simulink model "test_ads5296_fmca_r2_fmcb_r2_clk0"  (R2019a)
settings: Solver=FixedStepAuto  StartTime=0.0  StopTime=10.0  RelTol=1e-3
libraries: xbsIndex_r4 x3583, casper_library_misc x2, xps_library x1
(part 1 of 35)
settings Model: Creator=jackh  LastModifiedBy=jackh
settings DataIOCC: ReturnWorkspaceOutputs=off
settings DebuggingCC: PregeneratedLibrarySubsystemCodeDiagnostic=none  ArithmeticOperatorsInVariantConditions=warning
settings SFSimCC: SimUseLocalCustomCode=off
settings RTWCC: RTWUseLocalCustomCode=off

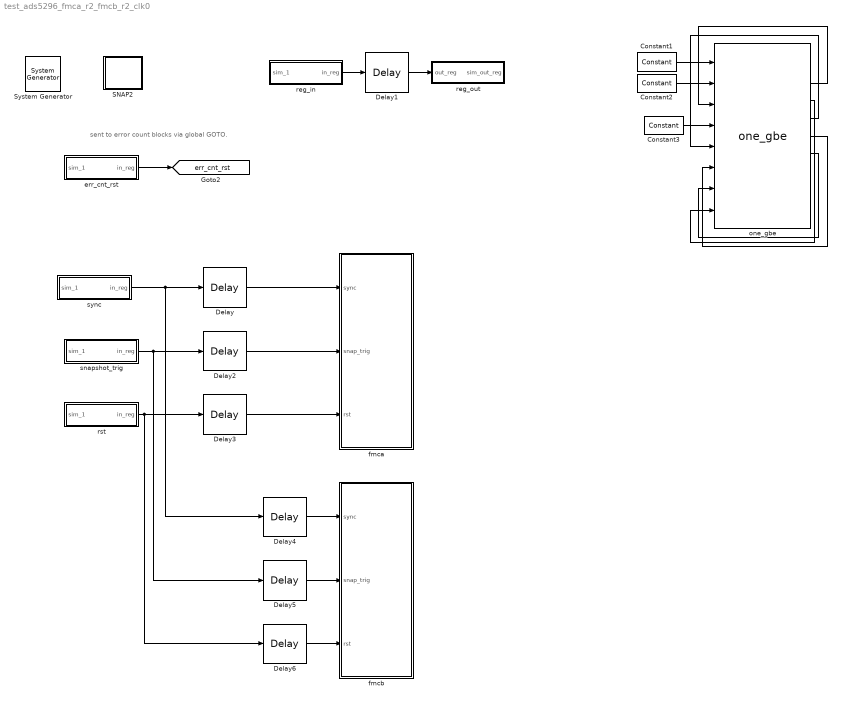
== system test_ads5296_fmca_r2_fmcb_r2_clk0 ==
  note: sent to error count blocks via global GOTO.
  " System Generator" : xbsIndex_r4/ System Generator  Tag=genX  xilinxfamily=kintexu  part=xcku115  speed=-2-e  package=flvf1924  synthesis_tool=XST  clock_wrapper=Clock Enables  directory=/home/jackh/src/caltech-lwa/test_models/ads5296_snap2_clkswitch_c/sysgen  proj_type=Vivado  Synth_file=Vivado Synthesis Defaults  Impl_file=Vivado Implementation Defaults  testbench=off  simulink_period=1  sysclk_period=5  dcm_input_clock_period=10  incr_netlist=off  trim_vbits=Everywhere in SubSystem  dbl_ovrd=According to Block Masks  core_generation=According to Block Masks  run_coregen=off  deprecated_control=off  eval_field=0  block_type=sysgen
  Constant1 : xbsIndex_r4/Constant  const=0  gui_display_data_type=Boolean  arith_type=Boolean  n_bits=16  bin_pt=14  preci_type=Single  exp_width=8  frac_width=24  explicit_period=on  period=1  equ=P=C  opselect=C  inp2=PCIN>>17  opr=+  inp1=P  carry=CIN  dbl_ovrd=off  block_type=constant
  Constant2 : xbsIndex_r4/Constant  const=0  gui_display_data_type=Boolean  arith_type=Boolean  n_bits=16  bin_pt=14  preci_type=Single  exp_width=8  frac_width=24  explicit_period=on  period=1  equ=P=C  opselect=C  inp2=PCIN>>17  opr=+  inp1=P  carry=CIN  dbl_ovrd=off  block_type=constant
  Constant3 : xbsIndex_r4/Constant  const=0  gui_display_data_type=Boolean  arith_type=Boolean  n_bits=16  bin_pt=14  preci_type=Single  exp_width=8  frac_width=24  explicit_period=on  period=1  equ=P=C  opselect=C  inp2=PCIN>>17  opr=+  inp1=P  carry=CIN  dbl_ovrd=off  block_type=constant
  Delay{,1..6} (7 alike) : xbsIndex_r4/Delay  rst=off  infoeditControl=Selection of Reset will increase slice count due to use of real FFs and instead of SRLs  en=off  latency=1  reg_retiming=off  dbl_ovrd=off  block_type=delay
  SNAP2 : Subsystem  Tag=xps:xsg  mask(xsg core config){hw_sys=SNAP2_v2:xcku115, clk_src=adc0_clk, clk_rate=200, use_microblaze=on, sample_period=1, synthesis_tool=XST}
      mask prompts: hw_sys "Hardware Platform"; clk_src "User IP Clock source"; clk_rate "User IP Clock Rate (MHz)"; use_microblaze "Use Microblaze controller?"; sample_period "Sample Period"; synthesis_tool "Synthesis Tool:"
      mask help:
      | The XSG Core Config block is used to configure the System Generator design
      | for the casper_xps toolflow. Settings here are used to configure the
      | Xilinx System Generator block parameters automatically, and control toolflow
      | script  execution. It needs to be at the top level of all designs being compiled
      | with the casper_xps toolflow.
      mask init:
      | xps_xsg_snap2_conf_mask;
      mask Help: eval('xlWeb([getenv(''MLIB_ROOT''), ''\doc\html\sys_xsg_core_config\sys_xsg_core_config.html''])')
      mask TypeOptions hw_sys: SNAP2_v1:xcku115 | SNAP2_v2:xcku115
      mask TypeOptions clk_src: sys_clk | clk_250MHz | adc0_clk | adc1_clk
      mask TypeOptions synthesis_tool: Leonardo Spectrum | Synplify | Synplify Pro | XST
      mask Display: fprintf(['SNAP2']);
  err_cnt_rst : Subsystem  Tag=xps:sw_reg  AncestorBlock=xps_library/Memory/software_register  mask(swreg){io_dir=From Processor, io_delay=0, init_val=0, sample_period=1, names=reg, bitwidths=1, bin_pts=0, arith_types=2, sim_port=on, show_format=on}
      mask prompts: io_dir "I/O direction"; io_delay "I/O delay"; init_val "Initial Value"; sample_period "Sample period"; names "Bitfield names [msb...lsb]"; bitwidths "Bitfield widths"; bin_pts "Bitfield binary pts"; arith_types "Bitfield types, ufix=0, fix=1, bool=2"; sim_port "Provide sim input/output?"; show_format "Print format string?"
      mask help: A 32-bit software-accessible register. Can be divided into bitfields of varying widths and types using the fields in the block mask.
      mask init:
      | swreg_init(gcb)
      settings: AttributesFormatString=1input:b = 1 bits
      mask TypeOptions io_dir: To Processor | From Processor
      mask Callback io_dir:
      | mask_enables = get_param(gcb, 'MaskEnables');
      | mask_names = get_param(gcb, 'MaskNames');
      | if strcmp(get_param(gcb, 'io_dir'), 'To Processor'),
      |     mask_enables{ismember(mask_names, 'sample_period')} = 'off';
      | else
      |     mask_enables{ismember(mask_names, 'sample_period')} = 'on';
      | end
      | set_param(gcb, 'MaskEnables', mask_enables);
      mask DialogControl ParameterTabVar0 Prompt: Setup
  fmca : Subsystem  mask{fmc_port=0, fmc_clock=0, board_version=2}
      mask prompts: fmc_port "FMC port"; fmc_clock "Use clock from which FMC"; board_version "Board version"
  fmcb : Subsystem  mask{fmc_port=1, fmc_clock=0, board_version=2}
      mask prompts: fmc_port "FMC port"; fmc_clock "Use clock from which FMC"; board_version "Board version"
  one_gbe : xps_library/IO/one_gbe  Tag=xps:onegbe  local_en=on  dis_cpu_rx=off  dis_cpu_tx=off  cpu_promiscuous=on  local_mac=hex2dec('123456789abc')  local_ip=hex2dec('c0a8290a')  local_port=4321  local_gateway=1
      settings: SourceProductName=CASPER XPS Blockset
  reg_in : Subsystem  Tag=xps:sw_reg  AncestorBlock=xps_library/Memory/software_register  mask(swreg){io_dir=From Processor, io_delay=0, init_val=0, sample_period=1, names=reg, bitwidths=10, bin_pts=9, arith_types=1, sim_port=on, show_format=on}
      mask prompts: io_dir "I/O direction"; io_delay "I/O delay"; init_val "Initial Value"; sample_period "Sample period"; names "Bitfield names [msb...lsb]"; bitwidths "Bitfield widths"; bin_pts "Bitfield binary pts"; arith_types "Bitfield types, ufix=0, fix=1, bool=2"; sim_port "Provide sim input/output?"; show_format "Print format string?"
      mask help: A 32-bit software-accessible register. Can be divided into bitfields of varying widths and types using the fields in the block mask.
      mask init:
      | swreg_init(gcb)
      settings: AttributesFormatString=1input:f10.9 = 10 bits
      mask TypeOptions io_dir: To Processor | From Processor
      mask Callback io_dir:
      | mask_enables = get_param(gcb, 'MaskEnables');
      | mask_names = get_param(gcb, 'MaskNames');
      | if strcmp(get_param(gcb, 'io_dir'), 'To Processor'),
      |     mask_enables{ismember(mask_names, 'sample_period')} = 'off';
      | else
      |     mask_enables{ismember(mask_names, 'sample_period')} = 'on';
      | end
      | set_param(gcb, 'MaskEnables', mask_enables);
      mask DialogControl ParameterTabVar0 Prompt: Setup
  reg_out : Subsystem  Tag=xps:sw_reg  AncestorBlock=xps_library/Memory/software_register  mask(swreg){io_dir=To Processor, io_delay=0, init_val=0, sample_period=1, names=reg, bitwidths=10, bin_pts=9, arith_types=1, sim_port=on, show_format=on}
      mask prompts: io_dir "I/O direction"; io_delay "I/O delay"; init_val "Initial Value"; sample_period "Sample period"; names "Bitfield names [msb...lsb]"; bitwidths "Bitfield widths"; bin_pts "Bitfield binary pts"; arith_types "Bitfield types, ufix=0, fix=1, bool=2"; sim_port "Provide sim input/output?"; show_format "Print format string?"
      mask help: A 32-bit software-accessible register. Can be divided into bitfields of varying widths and types using the fields in the block mask.
      mask init:
      | swreg_init(gcb)
      settings: AttributesFormatString=1output:f10.9 = 10 bits
      mask TypeOptions io_dir: To Processor | From Processor
      mask Callback io_dir:
      | mask_enables = get_param(gcb, 'MaskEnables');
      | mask_names = get_param(gcb, 'MaskNames');
      | if strcmp(get_param(gcb, 'io_dir'), 'To Processor'),
      |     mask_enables{ismember(mask_names, 'sample_period')} = 'off';
      | else
      |     mask_enables{ismember(mask_names, 'sample_period')} = 'on';
      | end
      | set_param(gcb, 'MaskEnables', mask_enables);
      mask DialogControl ParameterTabVar0 Prompt: Setup
  rst : Subsystem  Tag=xps:sw_reg  AncestorBlock=xps_library/Memory/software_register  mask(swreg){io_dir=From Processor, io_delay=0, init_val=0, sample_period=1, names=reg, bitwidths=1, bin_pts=0, arith_types=2, sim_port=on, show_format=on}
      mask prompts: io_dir "I/O direction"; io_delay "I/O delay"; init_val "Initial Value"; sample_period "Sample period"; names "Bitfield names [msb...lsb]"; bitwidths "Bitfield widths"; bin_pts "Bitfield binary pts"; arith_types "Bitfield types, ufix=0, fix=1, bool=2"; sim_port "Provide sim input/output?"; show_format "Print format string?"
      mask help: A 32-bit software-accessible register. Can be divided into bitfields of varying widths and types using the fields in the block mask.
      mask init:
      | swreg_init(gcb)
      settings: AttributesFormatString=1input:b = 1 bits
      mask TypeOptions io_dir: To Processor | From Processor
      mask Callback io_dir:
      | mask_enables = get_param(gcb, 'MaskEnables');
      | mask_names = get_param(gcb, 'MaskNames');
      | if strcmp(get_param(gcb, 'io_dir'), 'To Processor'),
      |     mask_enables{ismember(mask_names, 'sample_period')} = 'off';
      | else
      |     mask_enables{ismember(mask_names, 'sample_period')} = 'on';
      | end
      | set_param(gcb, 'MaskEnables', mask_enables);
      mask DialogControl ParameterTabVar0 Prompt: Setup
  snapshot_trig : Subsystem  Tag=xps:sw_reg  AncestorBlock=xps_library/Memory/software_register  mask(swreg){io_dir=From Processor, io_delay=0, init_val=0, sample_period=1, names=reg, bitwidths=1, bin_pts=0, arith_types=2, sim_port=on, show_format=on}
      mask prompts: io_dir "I/O direction"; io_delay "I/O delay"; init_val "Initial Value"; sample_period "Sample period"; names "Bitfield names [msb...lsb]"; bitwidths "Bitfield widths"; bin_pts "Bitfield binary pts"; arith_types "Bitfield types, ufix=0, fix=1, bool=2"; sim_port "Provide sim input/output?"; show_format "Print format string?"
      mask help: A 32-bit software-accessible register. Can be divided into bitfields of varying widths and types using the fields in the block mask.
      mask init:
      | swreg_init(gcb)
      settings: AttributesFormatString=1input:b = 1 bits
      mask TypeOptions io_dir: To Processor | From Processor
      mask Callback io_dir:
      | mask_enables = get_param(gcb, 'MaskEnables');
      | mask_names = get_param(gcb, 'MaskNames');
      | if strcmp(get_param(gcb, 'io_dir'), 'To Processor'),
      |     mask_enables{ismember(mask_names, 'sample_period')} = 'off';
      | else
      |     mask_enables{ismember(mask_names, 'sample_period')} = 'on';
      | end
      | set_param(gcb, 'MaskEnables', mask_enables);
      mask DialogControl ParameterTabVar0 Prompt: Setup
  sync : Subsystem  Tag=xps:sw_reg  AncestorBlock=xps_library/Memory/software_register  mask(swreg){io_dir=From Processor, io_delay=0, init_val=0, sample_period=1, names=reg, bitwidths=1, bin_pts=0, arith_types=2, sim_port=on, show_format=on}
      mask prompts: io_dir "I/O direction"; io_delay "I/O delay"; init_val "Initial Value"; sample_period "Sample period"; names "Bitfield names [msb...lsb]"; bitwidths "Bitfield widths"; bin_pts "Bitfield binary pts"; arith_types "Bitfield types, ufix=0, fix=1, bool=2"; sim_port "Provide sim input/output?"; show_format "Print format string?"
      mask help: A 32-bit software-accessible register. Can be divided into bitfields of varying widths and types using the fields in the block mask.
      mask init:
      | swreg_init(gcb)
      settings: AttributesFormatString=1input:b = 1 bits
      mask TypeOptions io_dir: To Processor | From Processor
      mask Callback io_dir:
      | mask_enables = get_param(gcb, 'MaskEnables');
      | mask_names = get_param(gcb, 'MaskNames');
      | if strcmp(get_param(gcb, 'io_dir'), 'To Processor'),
      |     mask_enables{ismember(mask_names, 'sample_period')} = 'off';
      | else
      |     mask_enables{ismember(mask_names, 'sample_period')} = 'on';
      | end
      | set_param(gcb, 'MaskEnables', mask_enables);
      mask DialogControl ParameterTabVar0 Prompt: Setup
  tag scope: err_cnt_rst=global
  wires:
  reg_in/1(in_reg) -> Delay1/1
  Delay1/1 -> reg_out/1(out_reg)
  Constant1/1 -> one_gbe/1
  Constant2/1 -> one_gbe/2
  one_gbe/3 -> one_gbe/3
  Constant3/1 -> one_gbe/4
  one_gbe/5 -> one_gbe/5
  one_gbe/6 -> one_gbe/6
  one_gbe/7 -> one_gbe/7
  one_gbe/4 -> one_gbe/8
  err_cnt_rst/1(in_reg) -> [err_cnt_rst]
  sync/1(in_reg) -> Delay4/1, Delay/1
  snapshot_trig/1(in_reg) -> Delay5/1, Delay2/1
  rst/1(in_reg) -> Delay6/1, Delay3/1
  Delay/1 -> fmca/1(sync)
  Delay2/1 -> fmca/2(snap_trig)
  Delay3/1 -> fmca/3(rst)
  Delay4/1 -> fmcb/1(sync)
  Delay5/1 -> fmcb/2(snap_trig)
  Delay6/1 -> fmcb/3(rst)

== system test_ads5296_fmca_r2_fmcb_r2_clk0/SNAP2 ==

== system test_ads5296_fmca_r2_fmcb_r2_clk0/err_cnt_rst ==
  sim_1 : Inport
  convert1_1 : DataTypeConversion  OutDataTypeStr=fixdt('ufix1_En0')  LockScale=on
  convert2_1 : DataTypeConversion  OutDataTypeStr=fixdt('ufix1_En0')  ConvertRealWorld=Stored Integer (SI)  LockScale=on
  gain_1 : Gain
  io_delay : xbsIndex_r4/Delay  rst=off  infoeditControl=Selection of Reset will increase slice count due to use of real FFs and instead of SRLs  en=off  latency=0  reg_retiming=on  dbl_ovrd=off  block_type=delay
  slice_reg : xbsIndex_r4/Slice  nbits=1  boolean_output=on  mode=Lower Bit Location + Width  bit1=0  base1=MSB of Input  bit0=0  base0=LSB of Input  dbl_ovrd=off  block_type=slice
  test_ads5296_fmca_r2_fmcb_r2_clk0_err_cnt_rst_user_data_out : xbsIndex_r4/Gateway In  gui_display_data_type=Fixed-point  arith_type=Unsigned  n_bits=32  bin_pt=0  preci_type=Single  exp_width=8  frac_width=24  rows=1  columns=1  quantization="Round  (unbiased: +/- Inf)"  overflow=Saturate  period=1  UseAsADC=off  ADCChannel='1'  interface=None  automatic_assignment=on  address_offset=hex2dec('00')  intf_name=''  intf_description=''  default_value=0  timing_constraint=None  locs_specified=off  LOCs={}  io_standard={}  inherit_from_input=off  hdl_port=on  dbl_ovrd=off  block_type=gatewayin
  in_reg : Outport
  wires:
  test_ads5296_fmca_r2_fmcb_r2_clk0_err_cnt_rst_user_data_out/1 -> io_delay/1
  sim_1/1 -> convert1_1/1
  convert1_1/1 -> convert2_1/1
  convert2_1/1 -> gain_1/1
  gain_1/1 -> test_ads5296_fmca_r2_fmcb_r2_clk0_err_cnt_rst_user_data_out/1
  io_delay/1 -> slice_reg/1
  slice_reg/1 -> in_reg/1

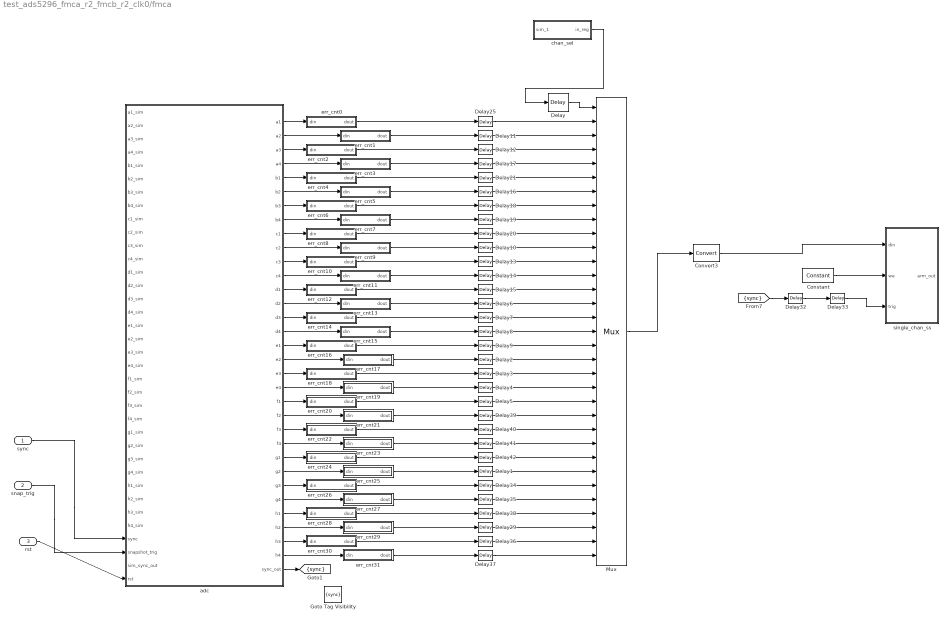
== system test_ads5296_fmca_r2_fmcb_r2_clk0/fmca ==
  sync : Inport
  snap_trig : Inport  Port=2
  rst : Inport  Port=3
  Constant : xbsIndex_r4/Constant  const=1  gui_display_data_type=Boolean  arith_type=Boolean  n_bits=16  bin_pt=14  preci_type=Single  exp_width=8  frac_width=24  explicit_period=on  period=1  equ=P=C  opselect=C  inp2=PCIN>>17  opr=+  inp1=P  carry=CIN  dbl_ovrd=off  block_type=constant
  Convert3 : xbsIndex_r4/Convert  gui_display_data_type=Fixed-point  arith_type="Signed  (2's comp)"  n_bits=16  bin_pt=15  float_type=Single  exp_bits=8  fraction_bits=24  quantization=Truncate  overflow=Wrap  en=off  latency=0  pipeline=off  dbl_ovrd=off  block_type=convert
  Delay : xbsIndex_r4/Delay  rst=off  infoeditControl=Selection of Reset will increase slice count due to use of real FFs and instead of SRLs  en=off  latency=6  reg_retiming=on  dbl_ovrd=off  block_type=delay
  Delay{1..21,25,29,32,34..42} (33 alike) : xbsIndex_r4/Delay  rst=off  infoeditControl=Selection of Reset will increase slice count due to use of real FFs and instead of SRLs  en=off  latency=2  reg_retiming=on  dbl_ovrd=off  block_type=delay
  Delay33 : xbsIndex_r4/Delay  rst=off  infoeditControl=Selection of Reset will increase slice count due to use of real FFs and instead of SRLs  en=off  latency=4  reg_retiming=on  dbl_ovrd=off  block_type=delay
  Goto Tag Visibility : GotoTagVisibility  GotoTag=sync
  Mux : xbsIndex_r4/Mux  inputs=32  en=off  latency=4  precision=Full  arith_type=Unsigned  n_bits=16  bin_pt=14  quantization=Truncate  overflow=Wrap  dbl_ovrd=off  block_type=mux
  adc : Subsystem  Tag=xps:ads5296x4  mask(ADS5296x4){board_count=2, sample_rate=200, port=fmc_port, clockport=fmc_clock, version=board_version}
      mask prompts: board_count "Number of quad-chip ADC Boards"; sample_rate "Sample Rate"; port "Which FMC port?"; clockport "Use clock from which FMC board?"; version "Which ADC board version?"
      mask help: 16-input ADC based on the TI ADS5296 chip.
      mask init:
      | % Only board_count is needed by init function
      | ads5296x4_init(gcb, ...
      |     'board_count', board_count);
      mask TypeOptions board_count: 1 | 2 | 3 | 4
  chan_sel : Subsystem  Tag=xps:sw_reg  AncestorBlock=xps_library/Memory/software_register  mask(swreg){io_dir=From Processor, io_delay=0, init_val=0, sample_period=1, names=reg, bitwidths=5, bin_pts=0, arith_types=0, sim_port=on, show_format=on}
      mask prompts: io_dir "I/O direction"; io_delay "I/O delay"; init_val "Initial Value"; sample_period "Sample period"; names "Bitfield names [msb...lsb]"; bitwidths "Bitfield widths"; bin_pts "Bitfield binary pts"; arith_types "Bitfield types, ufix=0, fix=1, bool=2"; sim_port "Provide sim input/output?"; show_format "Print format string?"
      mask help: A 32-bit software-accessible register. Can be divided into bitfields of varying widths and types using the fields in the block mask.
      mask init:
      | swreg_init(gcb)
      settings: AttributesFormatString=1input:uf5.0 = 5 bits
      mask TypeOptions io_dir: To Processor | From Processor
      mask Callback io_dir:
      | mask_enables = get_param(gcb, 'MaskEnables');
      | mask_names = get_param(gcb, 'MaskNames');
      | if strcmp(get_param(gcb, 'io_dir'), 'To Processor'),
      |     mask_enables{ismember(mask_names, 'sample_period')} = 'off';
      | else
      |     mask_enables{ismember(mask_names, 'sample_period')} = 'on';
      | end
      | set_param(gcb, 'MaskEnables', mask_enables);
      mask DialogControl ParameterTabVar0 Prompt: Setup
  err_cnt0 : Subsystem  VariantControl=Variant1
  err_cnt1 : Subsystem  VariantControl=Variant1
  err_cnt10 : Subsystem  VariantControl=Variant1
  err_cnt11 : Subsystem  VariantControl=Variant1
  err_cnt12 : Subsystem  VariantControl=Variant1
  err_cnt13 : Subsystem  VariantControl=Variant1
  err_cnt14 : Subsystem  VariantControl=Variant1
  err_cnt15 : Subsystem  VariantControl=Variant1
  err_cnt16 : Subsystem  VariantControl=Variant1
  err_cnt17 : Subsystem  VariantControl=Variant1
  err_cnt18 : Subsystem  VariantControl=Variant1
  err_cnt19 : Subsystem  VariantControl=Variant1
  err_cnt2 : Subsystem  VariantControl=Variant1
  err_cnt20 : Subsystem  VariantControl=Variant1
  err_cnt21 : Subsystem  VariantControl=Variant1
  err_cnt22 : Subsystem  VariantControl=Variant1
  err_cnt23 : Subsystem  VariantControl=Variant1
  err_cnt24 : Subsystem  VariantControl=Variant1
  err_cnt25 : Subsystem  VariantControl=Variant1
  err_cnt26 : Subsystem  VariantControl=Variant1
  err_cnt27 : Subsystem  VariantControl=Variant1
  err_cnt28 : Subsystem  VariantControl=Variant1
  err_cnt29 : Subsystem  VariantControl=Variant1
  err_cnt3 : Subsystem  VariantControl=Variant1
  err_cnt30 : Subsystem  VariantControl=Variant1
  err_cnt31 : Subsystem  VariantControl=Variant1
  err_cnt4 : Subsystem  VariantControl=Variant1
  err_cnt5 : Subsystem  VariantControl=Variant1
  err_cnt6 : Subsystem  VariantControl=Variant1
  err_cnt7 : Subsystem  VariantControl=Variant1
  err_cnt8 : Subsystem  VariantControl=Variant1
  err_cnt9 : Subsystem  VariantControl=Variant1
  single_chan_ss : Subsystem  Tag=casper:snapshot  AncestorBlock=casper_library_scopes/snapshot  mask(snapshot){storage=bram, dram_dimm=2, dram_clock=250, nsamples=16, data_width=16, offset=off, circap=off, value=off, ext_arm=off, ext_circ=off, provide_outputs=on, use_dsp48=off}
      mask prompts: storage "Storage medium"; dram_dimm "DRAM dimm"; dram_clock "DRAM clock rate"; nsamples "Number of Samples (2^?)"; data_width "Data width"; offset "Start delay support"; circap "Circular capture support"; value "Extra value capture support"; ext_arm "External arm support"; ext_circ "External circular capture support"; provide_outputs "Provide outputs"; use_dsp48 "Use DSP48s to implement counters"
      mask help:
      | Standard snap block, but with the following optional extras;
      |  1) Optionally delay the fabric trigger by a user-specified number of valids.
      |  2) Capture continuously after a trigger until a stop pulse is received. Data is captured into BRAM continuously, with old data being overwritten until a stop command is received. Then stop capturing when memory is filled. This enables you to get some data before and some data after the stop pulse. Use the 'tr_en_cnt' register to determine where you are in your vector. 'Addr' register's MSb now indicates 'busy capturing'.
      |  3) Optionally capture a value on an input port to a register at the same time as the first data sample.
      |  4) Implement counters using DSP48Es to save resources.
      mask init:
      | snapshot_init(gcb, ...
      |     'storage', storage, ...
      |     'dram_dimm', dram_dimm, ...
      |     'dram_clock', dram_clock, ...
      |     'nsamples', nsamples, ...
      |     'data_width', data_width, ...
      |     'offset', offset, ...
      |     'circap', circap, ...
      |     'value', value, ...
      |     'ext_arm', ext_arm, ...
      |     'ext_circ', ext_circ, ...
      |     'provide_outputs', 'off', ...
      |     'use_dsp48', use_dsp48);
      settings: AttributesFormatString=|
      | 16 wide, 65536 deep
      | debugID: 35264124
      mask TypeOptions storage: bram | dram
      mask Callback storage: snapshot_callback();
      mask TypeOptions dram_dimm: 1 | 2 | 3 | 4
      mask TypeOptions dram_clock: 200 | 250 | 266 | 300 | 333
      mask TypeOptions data_width: 8 | 16 | 32 | 64 | 128
  tag scope: sync=scoped
  wires:
  adc/16(d4) -> err_cnt15/1(din)
  adc/13(d1) -> err_cnt12/1(din)
  snap_trig/1 -> adc/34(snapshot_trig)
  adc/24(f4) -> err_cnt23/1(din)
  adc/2(a2) -> err_cnt1/1(din)
  adc/1(a1) -> err_cnt0/1(din)
  adc/23(f3) -> err_cnt22/1(din)
  Delay32/1 -> Delay33/1
  adc/4(a4) -> err_cnt3/1(din)
  adc/31(h3) -> err_cnt30/1(din)
  adc/27(g3) -> err_cnt26/1(din)
  adc/6(b2) -> err_cnt5/1(din)
  Mux/1 -> Convert3/1
  ? -> adc/35(sim_sync_out)
  adc/3(a3) -> err_cnt2/1(din)
  Delay36/1 -> Mux/32
  adc/32(h4) -> err_cnt31/1(din)
  Convert3/1 -> single_chan_ss/1(din)
  adc/33(sync_out) -> [sync]
  adc/5(b1) -> err_cnt4/1(din)
  adc/25(g1) -> err_cnt24/1(din)
  adc/18(e2) -> err_cnt17/1(din)
  adc/8(b4) -> err_cnt7/1(din)
  adc/10(c2) -> err_cnt9/1(din)
  Constant/1 -> single_chan_ss/2(we)
  Delay29/1 -> Mux/31
  adc/20(e4) -> err_cnt19/1(din)
  Delay37/1 -> Mux/33
  chan_sel/1(in_reg) -> Delay/1
  adc/12(c4) -> err_cnt11/1(din)
  rst/1 -> adc/36(rst)
  adc/26(g2) -> err_cnt25/1(din)
  sync/1 -> adc/33(sync)
  adc/14(d2) -> err_cnt13/1(din)
  adc/11(c3) -> err_cnt10/1(din)
  [sync] -> Delay32/1
  adc/22(f2) -> err_cnt21/1(din)
  adc/7(b3) -> err_cnt6/1(din)
  adc/29(h1) -> err_cnt28/1(din)
  adc/19(e3) -> err_cnt18/1(din)
  adc/15(d3) -> err_cnt14/1(din)
  adc/9(c1) -> err_cnt8/1(din)
  Delay/1 -> Mux/1
  adc/21(f1) -> err_cnt20/1(din)
  adc/30(h2) -> err_cnt29/1(din)
  adc/28(g4) -> err_cnt27/1(din)
  Delay33/1 -> single_chan_ss/3(trig)
  err_cnt31/1(dout) -> Delay37/1
  adc/17(e1) -> err_cnt16/1(din)
  err_cnt29/1(dout) -> Delay29/1
  err_cnt30/1(dout) -> Delay36/1
  err_cnt26/1(dout) -> Delay34/1
  err_cnt25/1(dout) -> Delay1/1
  err_cnt27/1(dout) -> Delay35/1
  err_cnt28/1(dout) -> Delay38/1
  err_cnt24/1(dout) -> Delay42/1
  err_cnt23/1(dout) -> Delay41/1
  err_cnt21/1(dout) -> Delay39/1
  err_cnt22/1(dout) -> Delay40/1
  err_cnt14/1(dout) -> Delay7/1
  err_cnt13/1(dout) -> Delay6/1
  err_cnt15/1(dout) -> Delay8/1
  err_cnt16/1(dout) -> Delay9/1
  err_cnt20/1(dout) -> Delay5/1
  err_cnt19/1(dout) -> Delay4/1
  err_cnt17/1(dout) -> Delay2/1
  err_cnt18/1(dout) -> Delay3/1
  err_cnt2/1(dout) -> Delay12/1
  err_cnt1/1(dout) -> Delay11/1
  err_cnt3/1(dout) -> Delay17/1
  err_cnt4/1(dout) -> Delay21/1
  err_cnt0/1(dout) -> Delay25/1
  err_cnt6/1(dout) -> Delay18/1
  err_cnt5/1(dout) -> Delay16/1
  err_cnt7/1(dout) -> Delay19/1
  err_cnt8/1(dout) -> Delay20/1
  err_cnt12/1(dout) -> Delay15/1
  err_cnt11/1(dout) -> Delay14/1
  err_cnt9/1(dout) -> Delay10/1
  err_cnt10/1(dout) -> Delay13/1
  Delay25/1 -> Mux/2
  Delay11/1 -> Mux/3
  Delay12/1 -> Mux/4
  Delay17/1 -> Mux/5
  Delay21/1 -> Mux/6
  Delay16/1 -> Mux/7
  Delay18/1 -> Mux/8
  Delay19/1 -> Mux/9
  Delay20/1 -> Mux/10
  Delay10/1 -> Mux/11
  Delay13/1 -> Mux/12
  Delay14/1 -> Mux/13
  Delay15/1 -> Mux/14
  Delay6/1 -> Mux/15
  Delay7/1 -> Mux/16
  Delay8/1 -> Mux/17
  Delay9/1 -> Mux/18
  Delay2/1 -> Mux/19
  Delay3/1 -> Mux/20
  Delay4/1 -> Mux/21
  Delay5/1 -> Mux/22
  Delay39/1 -> Mux/23
  Delay40/1 -> Mux/24
  Delay41/1 -> Mux/25
  Delay42/1 -> Mux/26
  Delay1/1 -> Mux/27
  Delay34/1 -> Mux/28
  Delay35/1 -> Mux/29
  Delay38/1 -> Mux/30

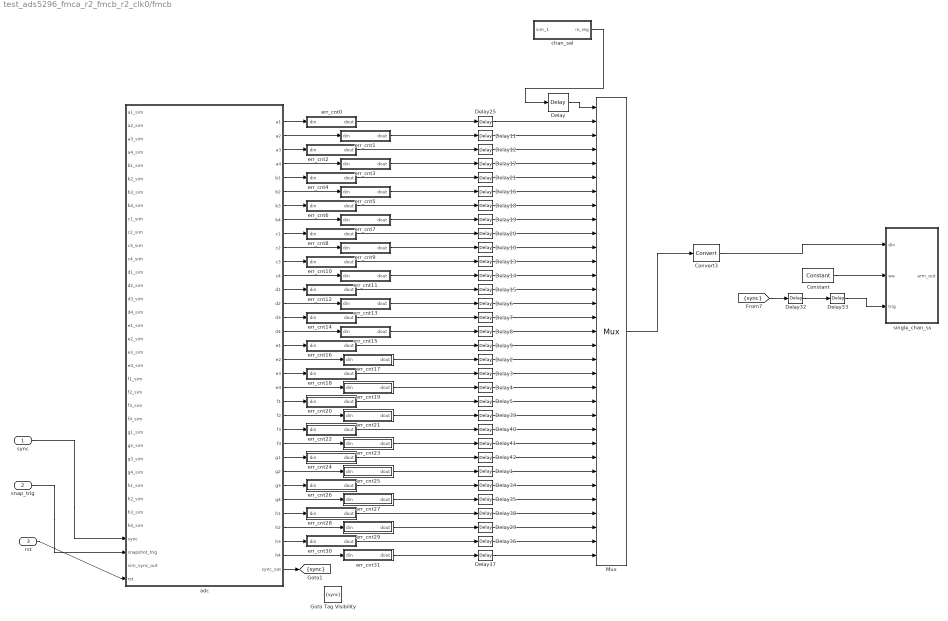
== system test_ads5296_fmca_r2_fmcb_r2_clk0/fmcb ==
  sync : Inport
  snap_trig : Inport  Port=2
  rst : Inport  Port=3
  Constant : xbsIndex_r4/Constant  const=1  gui_display_data_type=Boolean  arith_type=Boolean  n_bits=16  bin_pt=14  preci_type=Single  exp_width=8  frac_width=24  explicit_period=on  period=1  equ=P=C  opselect=C  inp2=PCIN>>17  opr=+  inp1=P  carry=CIN  dbl_ovrd=off  block_type=constant
  Convert3 : xbsIndex_r4/Convert  gui_display_data_type=Fixed-point  arith_type="Signed  (2's comp)"  n_bits=16  bin_pt=15  float_type=Single  exp_bits=8  fraction_bits=24  quantization=Truncate  overflow=Wrap  en=off  latency=0  pipeline=off  dbl_ovrd=off  block_type=convert
  Delay : xbsIndex_r4/Delay  rst=off  infoeditControl=Selection of Reset will increase slice count due to use of real FFs and instead of SRLs  en=off  latency=6  reg_retiming=on  dbl_ovrd=off  block_type=delay
  Delay{1..21,25,29,32,34..42} (33 alike) : xbsIndex_r4/Delay  rst=off  infoeditControl=Selection of Reset will increase slice count due to use of real FFs and instead of SRLs  en=off  latency=2  reg_retiming=on  dbl_ovrd=off  block_type=delay
  Delay33 : xbsIndex_r4/Delay  rst=off  infoeditControl=Selection of Reset will increase slice count due to use of real FFs and instead of SRLs  en=off  latency=4  reg_retiming=on  dbl_ovrd=off  block_type=delay
  Goto Tag Visibility : GotoTagVisibility  GotoTag=sync
  Mux : xbsIndex_r4/Mux  inputs=32  en=off  latency=4  precision=Full  arith_type=Unsigned  n_bits=16  bin_pt=14  quantization=Truncate  overflow=Wrap  dbl_ovrd=off  block_type=mux
  adc : Subsystem  Tag=xps:ads5296x4  mask(ADS5296x4){board_count=2, sample_rate=200, port=fmc_port, clockport=fmc_clock, version=board_version}
      mask prompts: board_count "Number of quad-chip ADC Boards"; sample_rate "Sample Rate"; port "Which FMC port?"; clockport "Use clock from which FMC board?"; version "Which ADC board version?"
      mask help: 16-input ADC based on the TI ADS5296 chip.
      mask init:
      | % Only board_count is needed by init function
      | ads5296x4_init(gcb, ...
      |     'board_count', board_count);
      mask TypeOptions board_count: 1 | 2 | 3 | 4
  chan_sel : Subsystem  Tag=xps:sw_reg  AncestorBlock=xps_library/Memory/software_register  mask(swreg){io_dir=From Processor, io_delay=0, init_val=0, sample_period=1, names=reg, bitwidths=5, bin_pts=0, arith_types=0, sim_port=on, show_format=on}
      mask prompts: io_dir "I/O direction"; io_delay "I/O delay"; init_val "Initial Value"; sample_period "Sample period"; names "Bitfield names [msb...lsb]"; bitwidths "Bitfield widths"; bin_pts "Bitfield binary pts"; arith_types "Bitfield types, ufix=0, fix=1, bool=2"; sim_port "Provide sim input/output?"; show_format "Print format string?"
      mask help: A 32-bit software-accessible register. Can be divided into bitfields of varying widths and types using the fields in the block mask.
      mask init:
      | swreg_init(gcb)
      settings: AttributesFormatString=1input:uf5.0 = 5 bits
      mask TypeOptions io_dir: To Processor | From Processor
      mask Callback io_dir:
      | mask_enables = get_param(gcb, 'MaskEnables');
      | mask_names = get_param(gcb, 'MaskNames');
      | if strcmp(get_param(gcb, 'io_dir'), 'To Processor'),
      |     mask_enables{ismember(mask_names, 'sample_period')} = 'off';
      | else
      |     mask_enables{ismember(mask_names, 'sample_period')} = 'on';
      | end
      | set_param(gcb, 'MaskEnables', mask_enables);
      mask DialogControl ParameterTabVar0 Prompt: Setup
  err_cnt0 : Subsystem  VariantControl=Variant1
  err_cnt1 : Subsystem  VariantControl=Variant1
  err_cnt10 : Subsystem  VariantControl=Variant1
  err_cnt11 : Subsystem  VariantControl=Variant1
  err_cnt12 : Subsystem  VariantControl=Variant1
  err_cnt13 : Subsystem  VariantControl=Variant1
  err_cnt14 : Subsystem  VariantControl=Variant1
  err_cnt15 : Subsystem  VariantControl=Variant1
  err_cnt16 : Subsystem  VariantControl=Variant1
  err_cnt17 : Subsystem  VariantControl=Variant1
  err_cnt18 : Subsystem  VariantControl=Variant1
  err_cnt19 : Subsystem  VariantControl=Variant1
  err_cnt2 : Subsystem  VariantControl=Variant1
  err_cnt20 : Subsystem  VariantControl=Variant1
  err_cnt21 : Subsystem  VariantControl=Variant1
  err_cnt22 : Subsystem  VariantControl=Variant1
  err_cnt23 : Subsystem  VariantControl=Variant1
  err_cnt24 : Subsystem  VariantControl=Variant1
  err_cnt25 : Subsystem  VariantControl=Variant1
  err_cnt26 : Subsystem  VariantControl=Variant1
  err_cnt27 : Subsystem  VariantControl=Variant1
  err_cnt28 : Subsystem  VariantControl=Variant1
  err_cnt29 : Subsystem  VariantControl=Variant1
  err_cnt3 : Subsystem  VariantControl=Variant1
  err_cnt30 : Subsystem  VariantControl=Variant1
  err_cnt31 : Subsystem  VariantControl=Variant1
  err_cnt4 : Subsystem  VariantControl=Variant1
  err_cnt5 : Subsystem  VariantControl=Variant1
  err_cnt6 : Subsystem  VariantControl=Variant1
  err_cnt7 : Subsystem  VariantControl=Variant1
  err_cnt8 : Subsystem  VariantControl=Variant1
  err_cnt9 : Subsystem  VariantControl=Variant1
  single_chan_ss : Subsystem  Tag=casper:snapshot  AncestorBlock=casper_library_scopes/snapshot  mask(snapshot){storage=bram, dram_dimm=2, dram_clock=250, nsamples=16, data_width=16, offset=off, circap=off, value=off, ext_arm=off, ext_circ=off, provide_outputs=on, use_dsp48=off}
      mask prompts: storage "Storage medium"; dram_dimm "DRAM dimm"; dram_clock "DRAM clock rate"; nsamples "Number of Samples (2^?)"; data_width "Data width"; offset "Start delay support"; circap "Circular capture support"; value "Extra value capture support"; ext_arm "External arm support"; ext_circ "External circular capture support"; provide_outputs "Provide outputs"; use_dsp48 "Use DSP48s to implement counters"
      mask help:
      | Standard snap block, but with the following optional extras;
      |  1) Optionally delay the fabric trigger by a user-specified number of valids.
      |  2) Capture continuously after a trigger until a stop pulse is received. Data is captured into BRAM continuously, with old data being overwritten until a stop command is received. Then stop capturing when memory is filled. This enables you to get some data before and some data after the stop pulse. Use the 'tr_en_cnt' register to determine where you are in your vector. 'Addr' register's MSb now indicates 'busy capturing'.
      |  3) Optionally capture a value on an input port to a register at the same time as the first data sample.
      |  4) Implement counters using DSP48Es to save resources.
      mask init: same as test_ads5296_fmca_r2_fmcb_r2_clk0/fmca/single_chan_ss
      settings: AttributesFormatString=|
      | 16 wide, 65536 deep
      | debugID: 35264124
      mask TypeOptions storage: bram | dram
      mask Callback storage: snapshot_callback();
      mask TypeOptions dram_dimm: 1 | 2 | 3 | 4
      mask TypeOptions dram_clock: 200 | 250 | 266 | 300 | 333
      mask TypeOptions data_width: 8 | 16 | 32 | 64 | 128
  tag scope: sync=scoped
  wires:
  Delay38/1 -> Mux/30
  Delay35/1 -> Mux/29
  Delay34/1 -> Mux/28
  Delay1/1 -> Mux/27
  Delay42/1 -> Mux/26
  Delay41/1 -> Mux/25
  Delay40/1 -> Mux/24
  Delay39/1 -> Mux/23
  Delay5/1 -> Mux/22
  Delay4/1 -> Mux/21
  Delay3/1 -> Mux/20
  Delay2/1 -> Mux/19
  Delay9/1 -> Mux/18
  Delay8/1 -> Mux/17
  Delay7/1 -> Mux/16
  Delay6/1 -> Mux/15
  Delay15/1 -> Mux/14
  Delay14/1 -> Mux/13
  Delay13/1 -> Mux/12
  Delay10/1 -> Mux/11
  Delay20/1 -> Mux/10
  Delay19/1 -> Mux/9
  Delay18/1 -> Mux/8
  Delay16/1 -> Mux/7
  Delay21/1 -> Mux/6
  Delay17/1 -> Mux/5
  Delay12/1 -> Mux/4
  Delay11/1 -> Mux/3
  Delay25/1 -> Mux/2
  err_cnt10/1(dout) -> Delay13/1
  err_cnt9/1(dout) -> Delay10/1
  err_cnt11/1(dout) -> Delay14/1
  err_cnt12/1(dout) -> Delay15/1
  err_cnt8/1(dout) -> Delay20/1
  err_cnt7/1(dout) -> Delay19/1
  err_cnt5/1(dout) -> Delay16/1
  err_cnt6/1(dout) -> Delay18/1
  err_cnt0/1(dout) -> Delay25/1
  err_cnt4/1(dout) -> Delay21/1
  err_cnt3/1(dout) -> Delay17/1
  err_cnt1/1(dout) -> Delay11/1
  err_cnt2/1(dout) -> Delay12/1
  err_cnt18/1(dout) -> Delay3/1
  err_cnt17/1(dout) -> Delay2/1
  err_cnt19/1(dout) -> Delay4/1
  err_cnt20/1(dout) -> Delay5/1
  err_cnt16/1(dout) -> Delay9/1
  err_cnt15/1(dout) -> Delay8/1
  err_cnt13/1(dout) -> Delay6/1
  err_cnt14/1(dout) -> Delay7/1
  err_cnt22/1(dout) -> Delay40/1
  err_cnt21/1(dout) -> Delay39/1
  err_cnt23/1(dout) -> Delay41/1
  err_cnt24/1(dout) -> Delay42/1
  err_cnt28/1(dout) -> Delay38/1
  err_cnt27/1(dout) -> Delay35/1
  err_cnt25/1(dout) -> Delay1/1
  err_cnt26/1(dout) -> Delay34/1
  err_cnt30/1(dout) -> Delay36/1
  err_cnt29/1(dout) -> Delay29/1
  adc/17(e1) -> err_cnt16/1(din)
  err_cnt31/1(dout) -> Delay37/1
  Delay33/1 -> single_chan_ss/3(trig)
  adc/28(g4) -> err_cnt27/1(din)
  adc/30(h2) -> err_cnt29/1(din)
  adc/21(f1) -> err_cnt20/1(din)
  Delay/1 -> Mux/1
  adc/9(c1) -> err_cnt8/1(din)
  adc/15(d3) -> err_cnt14/1(din)
  adc/19(e3) -> err_cnt18/1(din)
  adc/29(h1) -> err_cnt28/1(din)
  adc/7(b3) -> err_cnt6/1(din)
  adc/22(f2) -> err_cnt21/1(din)
  [sync] -> Delay32/1
  adc/11(c3) -> err_cnt10/1(din)
  adc/14(d2) -> err_cnt13/1(din)
  sync/1 -> adc/33(sync)
  adc/26(g2) -> err_cnt25/1(din)
  rst/1 -> adc/36(rst)
  adc/12(c4) -> err_cnt11/1(din)
  chan_sel/1(in_reg) -> Delay/1
  Delay37/1 -> Mux/33
  adc/20(e4) -> err_cnt19/1(din)
  Delay29/1 -> Mux/31
  Constant/1 -> single_chan_ss/2(we)
  adc/10(c2) -> err_cnt9/1(din)
  adc/8(b4) -> err_cnt7/1(din)
  adc/18(e2) -> err_cnt17/1(din)
  adc/25(g1) -> err_cnt24/1(din)
  adc/5(b1) -> err_cnt4/1(din)
  adc/33(sync_out) -> [sync]
  Convert3/1 -> single_chan_ss/1(din)
  adc/32(h4) -> err_cnt31/1(din)
  Delay36/1 -> Mux/32
  adc/3(a3) -> err_cnt2/1(din)
  ? -> adc/35(sim_sync_out)
  Mux/1 -> Convert3/1
  adc/6(b2) -> err_cnt5/1(din)
  adc/27(g3) -> err_cnt26/1(din)
  adc/31(h3) -> err_cnt30/1(din)
  adc/4(a4) -> err_cnt3/1(din)
  Delay32/1 -> Delay33/1
  adc/23(f3) -> err_cnt22/1(din)
  adc/1(a1) -> err_cnt0/1(din)
  adc/2(a2) -> err_cnt1/1(din)
  adc/24(f4) -> err_cnt23/1(din)
  snap_trig/1 -> adc/34(snapshot_trig)
  adc/13(d1) -> err_cnt12/1(din)
  adc/16(d4) -> err_cnt15/1(din)

== system test_ads5296_fmca_r2_fmcb_r2_clk0/reg_in ==
  sim_1 : Inport
  convert1_1 : DataTypeConversion  OutDataTypeStr=fixdt('ufix10_En9')  LockScale=on
  convert2_1 : DataTypeConversion  OutDataTypeStr=fixdt('ufix10_En0')  ConvertRealWorld=Stored Integer (SI)  LockScale=on
  gain_1 : Gain
  io_delay : xbsIndex_r4/Delay  rst=off  infoeditControl=Selection of Reset will increase slice count due to use of real FFs and instead of SRLs  en=off  latency=0  reg_retiming=on  dbl_ovrd=off  block_type=delay
  reint1 : xbsIndex_r4/Reinterpret  force_arith_type=on  arith_type="Signed  (2's comp)"  force_bin_pt=on  bin_pt=9  block_type=reinterpret
  slice_reg : xbsIndex_r4/Slice  nbits=10  boolean_output=off  mode=Lower Bit Location + Width  bit1=0  base1=MSB of Input  bit0=0  base0=LSB of Input  dbl_ovrd=off  block_type=slice
  test_ads5296_fmca_r2_fmcb_r2_clk0_reg_in_user_data_out : xbsIndex_r4/Gateway In  gui_display_data_type=Fixed-point  arith_type=Unsigned  n_bits=32  bin_pt=0  preci_type=Single  exp_width=8  frac_width=24  rows=1  columns=1  quantization="Round  (unbiased: +/- Inf)"  overflow=Saturate  period=1  UseAsADC=off  ADCChannel='1'  interface=None  automatic_assignment=on  address_offset=hex2dec('00')  intf_name=''  intf_description=''  default_value=0  timing_constraint=None  locs_specified=off  LOCs={}  io_standard={}  inherit_from_input=off  hdl_port=on  dbl_ovrd=off  block_type=gatewayin
  in_reg : Outport
  wires:
  test_ads5296_fmca_r2_fmcb_r2_clk0_reg_in_user_data_out/1 -> io_delay/1
  sim_1/1 -> convert1_1/1
  convert1_1/1 -> convert2_1/1
  convert2_1/1 -> gain_1/1
  gain_1/1 -> test_ads5296_fmca_r2_fmcb_r2_clk0_reg_in_user_data_out/1
  io_delay/1 -> slice_reg/1
  slice_reg/1 -> reint1/1
  reint1/1 -> in_reg/1

== system test_ads5296_fmca_r2_fmcb_r2_clk0/reg_out ==
  out_reg : Inport
  assert_reg : xbsIndex_r4/Assert  assert_type=on  type_source=Explicitly  gui_display_data_type=Fixed-point  arith_type="Signed  (2's comp)"  n_bits=10  bin_pt=9  preci_type=Single  exp_width=8  frac_width=24  assert_rate=off  rate_source=Explicitly  period=1  output_port=on  block_type=assert
  cast_gw : xbsIndex_r4/Convert  gui_display_data_type=Fixed-point  arith_type=Unsigned  n_bits=32  bin_pt=0  float_type=Single  exp_bits=8  fraction_bits=24  quantization=Truncate  overflow=Wrap  en=off  latency=1  pipeline=off  dbl_ovrd=off  block_type=convert
  io_delay : xbsIndex_r4/Delay  rst=off  infoeditControl=Selection of Reset will increase slice count due to use of real FFs and instead of SRLs  en=off  latency=0  reg_retiming=on  dbl_ovrd=off  block_type=delay
  reint1 : xbsIndex_r4/Reinterpret  force_arith_type=on  arith_type=Unsigned  force_bin_pt=on  bin_pt=0  block_type=reinterpret
  sim_out : Terminator
  sim_out_reg_gw : xbsIndex_r4/Gateway Out  inherit_from_input=off  hdl_port=off  rows=1  columns=1  UseAsDAC=off  DACChannel='1'  interface=None  automatic_assignment=on  address_offset=hex2dec('00')  intf_name=''  intf_description=''  timing_constraint=None  locs_specified=off  LOCs={}  io_standard={}  block_type=gatewayout
  sim_out_reg_sim_delay : xbsIndex_r4/Delay  rst=off  infoeditControl=Selection of Reset will increase slice count due to use of real FFs and instead of SRLs  en=off  latency=1  reg_retiming=on  dbl_ovrd=off  block_type=delay
  test_ads5296_fmca_r2_fmcb_r2_clk0_reg_out_user_data_in : xbsIndex_r4/Gateway Out  inherit_from_input=off  hdl_port=on  rows=1  columns=1  UseAsDAC=off  DACChannel='1'  interface=None  automatic_assignment=on  address_offset=hex2dec('00')  intf_name=''  intf_description=''  timing_constraint=None  locs_specified=off  LOCs={}  io_standard={}  block_type=gatewayout
  sim_out_reg : Outport
  wires:
  sim_out_reg_sim_delay/1 -> sim_out_reg_gw/1
  sim_out_reg_gw/1 -> sim_out_reg/1
  io_delay/1 -> cast_gw/1
  cast_gw/1 -> test_ads5296_fmca_r2_fmcb_r2_clk0_reg_out_user_data_in/1
  test_ads5296_fmca_r2_fmcb_r2_clk0_reg_out_user_data_in/1 -> sim_out/1
  out_reg/1 -> sim_out_reg_sim_delay/1, assert_reg/1
  assert_reg/1 -> reint1/1
  reint1/1 -> io_delay/1

== system test_ads5296_fmca_r2_fmcb_r2_clk0/rst ==
  sim_1 : Inport
  convert1_1 : DataTypeConversion  OutDataTypeStr=fixdt('ufix1_En0')  LockScale=on
  convert2_1 : DataTypeConversion  OutDataTypeStr=fixdt('ufix1_En0')  ConvertRealWorld=Stored Integer (SI)  LockScale=on
  gain_1 : Gain
  io_delay : xbsIndex_r4/Delay  rst=off  infoeditControl=Selection of Reset will increase slice count due to use of real FFs and instead of SRLs  en=off  latency=0  reg_retiming=on  dbl_ovrd=off  block_type=delay
  slice_reg : xbsIndex_r4/Slice  nbits=1  boolean_output=on  mode=Lower Bit Location + Width  bit1=0  base1=MSB of Input  bit0=0  base0=LSB of Input  dbl_ovrd=off  block_type=slice
  test_ads5296_fmca_r2_fmcb_r2_clk0_rst_user_data_out : xbsIndex_r4/Gateway In  gui_display_data_type=Fixed-point  arith_type=Unsigned  n_bits=32  bin_pt=0  preci_type=Single  exp_width=8  frac_width=24  rows=1  columns=1  quantization="Round  (unbiased: +/- Inf)"  overflow=Saturate  period=1  UseAsADC=off  ADCChannel='1'  interface=None  automatic_assignment=on  address_offset=hex2dec('00')  intf_name=''  intf_description=''  default_value=0  timing_constraint=None  locs_specified=off  LOCs={}  io_standard={}  inherit_from_input=off  hdl_port=on  dbl_ovrd=off  block_type=gatewayin
  in_reg : Outport
  wires:
  test_ads5296_fmca_r2_fmcb_r2_clk0_rst_user_data_out/1 -> io_delay/1
  sim_1/1 -> convert1_1/1
  convert1_1/1 -> convert2_1/1
  convert2_1/1 -> gain_1/1
  gain_1/1 -> test_ads5296_fmca_r2_fmcb_r2_clk0_rst_user_data_out/1
  io_delay/1 -> slice_reg/1
  slice_reg/1 -> in_reg/1

== system test_ads5296_fmca_r2_fmcb_r2_clk0/snapshot_trig ==
  sim_1 : Inport
  convert1_1 : DataTypeConversion  OutDataTypeStr=fixdt('ufix1_En0')  LockScale=on
  convert2_1 : DataTypeConversion  OutDataTypeStr=fixdt('ufix1_En0')  ConvertRealWorld=Stored Integer (SI)  LockScale=on
  gain_1 : Gain
  io_delay : xbsIndex_r4/Delay  rst=off  infoeditControl=Selection of Reset will increase slice count due to use of real FFs and instead of SRLs  en=off  latency=0  reg_retiming=on  dbl_ovrd=off  block_type=delay
  slice_reg : xbsIndex_r4/Slice  nbits=1  boolean_output=on  mode=Lower Bit Location + Width  bit1=0  base1=MSB of Input  bit0=0  base0=LSB of Input  dbl_ovrd=off  block_type=slice
  test_ads5296_fmca_r2_fmcb_r2_clk0_snapshot_trig_user_data_out : xbsIndex_r4/Gateway In  gui_display_data_type=Fixed-point  arith_type=Unsigned  n_bits=32  bin_pt=0  preci_type=Single  exp_width=8  frac_width=24  rows=1  columns=1  quantization="Round  (unbiased: +/- Inf)"  overflow=Saturate  period=1  UseAsADC=off  ADCChannel='1'  interface=None  automatic_assignment=on  address_offset=hex2dec('00')  intf_name=''  intf_description=''  default_value=0  timing_constraint=None  locs_specified=off  LOCs={}  io_standard={}  inherit_from_input=off  hdl_port=on  dbl_ovrd=off  block_type=gatewayin
  in_reg : Outport
  wires:
  test_ads5296_fmca_r2_fmcb_r2_clk0_snapshot_trig_user_data_out/1 -> io_delay/1
  sim_1/1 -> convert1_1/1
  convert1_1/1 -> convert2_1/1
  convert2_1/1 -> gain_1/1
  gain_1/1 -> test_ads5296_fmca_r2_fmcb_r2_clk0_snapshot_trig_user_data_out/1
  io_delay/1 -> slice_reg/1
  slice_reg/1 -> in_reg/1

== system test_ads5296_fmca_r2_fmcb_r2_clk0/sync ==
  sim_1 : Inport
  convert1_1 : DataTypeConversion  OutDataTypeStr=fixdt('ufix1_En0')  LockScale=on
  convert2_1 : DataTypeConversion  OutDataTypeStr=fixdt('ufix1_En0')  ConvertRealWorld=Stored Integer (SI)  LockScale=on
  gain_1 : Gain
  io_delay : xbsIndex_r4/Delay  rst=off  infoeditControl=Selection of Reset will increase slice count due to use of real FFs and instead of SRLs  en=off  latency=0  reg_retiming=on  dbl_ovrd=off  block_type=delay
  slice_reg : xbsIndex_r4/Slice  nbits=1  boolean_output=on  mode=Lower Bit Location + Width  bit1=0  base1=MSB of Input  bit0=0  base0=LSB of Input  dbl_ovrd=off  block_type=slice
  test_ads5296_fmca_r2_fmcb_r2_clk0_sync_user_data_out : xbsIndex_r4/Gateway In  gui_display_data_type=Fixed-point  arith_type=Unsigned  n_bits=32  bin_pt=0  preci_type=Single  exp_width=8  frac_width=24  rows=1  columns=1  quantization="Round  (unbiased: +/- Inf)"  overflow=Saturate  period=1  UseAsADC=off  ADCChannel='1'  interface=None  automatic_assignment=on  address_offset=hex2dec('00')  intf_name=''  intf_description=''  default_value=0  timing_constraint=None  locs_specified=off  LOCs={}  io_standard={}  inherit_from_input=off  hdl_port=on  dbl_ovrd=off  block_type=gatewayin
  in_reg : Outport
  wires:
  test_ads5296_fmca_r2_fmcb_r2_clk0_sync_user_data_out/1 -> io_delay/1
  sim_1/1 -> convert1_1/1
  convert1_1/1 -> convert2_1/1
  convert2_1/1 -> gain_1/1
  gain_1/1 -> test_ads5296_fmca_r2_fmcb_r2_clk0_sync_user_data_out/1
  io_delay/1 -> slice_reg/1
  slice_reg/1 -> in_reg/1
